simulink model "parcial2tema1ejercicio5"  (R2021a)
settings: Solver=ode45  StartTime=0.0  StopTime=10.0  RelTol=1e-3  EnableMultiTasking=on
values from neighbouring files (symbols this model uses):
  C = 3  6  9 12 15    [tp1.m]    (also in tp3.m = FaC(F))
undefined symbols (not defined in the file or in its folder): none, Rec, SDTV, videoinput
libraries: visionconversions x1, imaqlib x1, visionanalysis x1
settings Model: Creator=eae  LastModifiedBy=ZeK005
settings SolverCC: AlgebraicLoopSolver=TrustRegion
settings DataIOCC: LimitDataPoints=on  SaveFormat=Array  ReturnWorkspaceOutputs=off
settings OptimizationCC: LifeSpan=inf
settings DebuggingCC: UnderspecifiedInitializationDetection=Classic  MergeDetectMultiDrivingBlocksExec=none  SolverPrmCheckMsg=warning  StateNameClashWarn=warning  SFUnexpectedBacktrackingDiag=warning  SFNoUnconditionalDefaultTransitionDiag=warning  SFExecutionAtInitializationDiag=none  SFMachineParentedDataDiag=warning  ArithmeticOperatorsInVariantConditions=warning
settings HardwareCC: ProdBitPerPointer=32  ProdBitPerSizeT=32  ProdBitPerPtrDiffT=32  ProdLargestAtomicFloat=None  ProdIntDivRoundTo=Undefined  ProdEndianess=Unspecified  ProdWordSize=32  ProdHWDeviceType=32-bit Generic
settings ModelReferenceCC: PropagateSignalLabelsOutOfModel=off
settings SFSimCC: SimUseLocalCustomCode=off  CustomCodeUndefinedFunction=UseInterfaceOnly
settings RTWCC: RTWUseLocalCustomCode=off
settings CodeAppCC: StateflowObjectComments=on
settings GRTTargetCC: TargetLangStandard=C89/C90 (ANSI)
settings ConfigComp: CovMetricSettings=dw  CovSaveCumulativeToWorkspaceVar=on  CovSaveSingleToWorkspaceVar=on  CovExternalEMLEnable=off

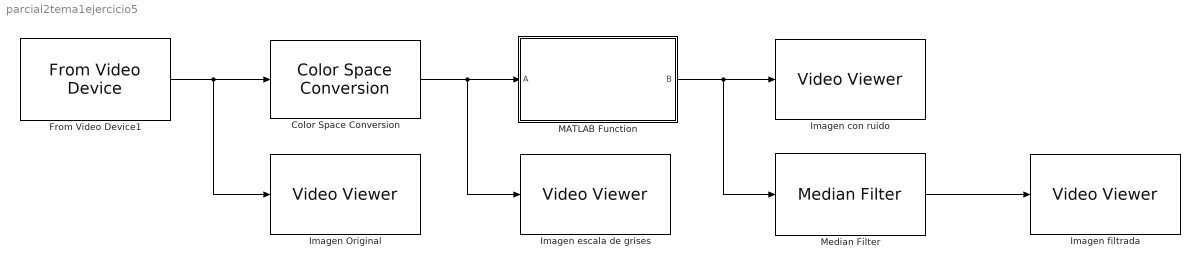
== system parcial2tema1ejercicio5 ==
  Color Space Conversion : visionconversions/Color Space  Conversion  conversion=Obsolete  conversionActive=R'G'B' to intensity  wp_str=D65  rec=Rec. 601 (SDTV)  sys=1125/60/2:1  imagePorts=One multidimensional signal
  From Video Device1 : imaqlib/From Video Device  DeviceMenu=winvideo 2 (OBS Virtual Camera)  Device=winvideo 2 (OBS Virtual Camera)  ObjConstructor=videoinput('winvideo', 2)  VideoFormatMenu=I420_640x360  VideoFormat=I420_640x360  VideoSource=input1  ROIPosition=[0 0 360 640]  EnableHWTrigger=off  TriggerConfiguration=none/none  SampleTime=1/30  OutputPortsMode=One multidimensional signal  DataType=single  CanDoHWTrigger=no  ReturnedColorSpace=rgb  BlockHandle=1851.0001  ROIWidth=640  ROIHeight=360  ROIColumn=0  ROIRow=0  EngXMLPath=C:\Program Files\Polyspace\R2021a\toolbox\imaq\imaq\private  DevXMLPath=C:\ProgramData\MATLAB\SupportPackages\R2021a\toolbox\imaq\supportpackages\genericvideo\adaptor\win64  EngLibPath=C:\Program Files\Polyspace\R2021a\toolbox\imaq\imaqblks\imaqmex\win64  ColorSpace=rgb  BayerSensorAlignment=grbg  ImaqMode=off
  Imagen Original : VideoViewer  FigPos=[50 416 410 300]
  Imagen con ruido : VideoViewer  FigPos=[1369 433 410 300]
  Imagen escala de grises : VideoViewer  FigPos=[90 899 410 300]
  Imagen filtrada : VideoViewer  FigPos=[1356 858 410 300]
  MATLAB Function : MATLAB Function  TreatAsAtomicUnit=on
  Median Filter : visionanalysis/Median Filter  nghbood=[3 3]  outSize=Same as input port I  padType=Constant  padSrc=Specify via dialog  padVal=0  roundingMode=Floor  overflowMode=off
      settings: SourceProductBaseCode=VP
  wires:
  From Video Device1/1 -> Imagen Original/1, Color Space Conversion/1
  Color Space Conversion/1 -> Imagen escala de grises/1, MATLAB Function/1(A)
  MATLAB Function/1(B) -> Median Filter/1, Imagen con ruido/1
  Median Filter/1 -> Imagen filtrada/1

== matlab function parcial2tema1ejercicio5/MATLAB Function ==
  data: A input; B output
function B = ruidopro(A)
%ruido
B=A;
%se obtiene el tamaño de la imagen
[m n]=size(A);
%Se distorcionan 300 puntos de la imagen con ruido sal
for v=1:10000
    % Se obtiene la posicion del pixel a distorsionar    
    x=round((m-1)*rand);
    y=round((n-1)*rand);
    % Se protege si el valor obtenido es cero
    if(x==0)
        x=1;
    end
    % Se protege si el valor obtenido es cero
    if(y==0)
        y=1;
    end
    %se distorsiona el pixel
    B(x,y)=1;
end
% Se distorsionan 300 puntos de la imagen con ruido pimienta 
for v=1:10000
    x=round((m-1)*rand);
    y=round((n-1)*rand);
    if(x==0)
        x=1;
    end
    if(y==0)
        y=1;
    end
    B(x,y)=0;
end
